simulink model "snb_bc"  (R2012b)
settings: Solver=FixedStepDiscrete  SolverMode=SingleTasking  StartTime=0.0  StopTime=10000  RelTol=1e-3
undefined symbols (not defined in the file): Down, pfb_coeff_gen_calc, Up
libraries: xbsIndex_r4 x19640, casper_library_misc x44, casper_library_delays x18, casper_library_communications x8, xps_library x3
(part 49 of 163)

== system snb_bc/mix_dec_fir/mixer/dds ==
  lo_const0 : Subsystem  AncestorBlock=casper_library_downconverter/lo_const  mask(lo_const){n_bits=10, phase=0}
      mask prompts: n_bits "Output Bitwidth"; phase "Phase (0 to 2*pi)"
      mask help:
      | Generates a complex constant associated with the
      | phase supplied as a parameter.
      mask init:
      | lo_const_init(gcb, ...
      |     'n_bits', n_bits, ...
      |     'phase', phase);
      mask Help: eval('xlWeb(''http://casper.berkeley.edu/wiki/Lo_const'')')
  lo_const1 : Subsystem  AncestorBlock=casper_library_downconverter/lo_const  mask(lo_const){n_bits=10, phase=1.5708}
      mask prompts: n_bits "Output Bitwidth"; phase "Phase (0 to 2*pi)"
      mask help:
      | Generates a complex constant associated with the
      | phase supplied as a parameter.
      mask init:
      | lo_const_init(gcb, ...
      |     'n_bits', n_bits, ...
      |     'phase', phase);
      mask Help: eval('xlWeb(''http://casper.berkeley.edu/wiki/Lo_const'')')
  lo_const2 : Subsystem  AncestorBlock=casper_library_downconverter/lo_const  mask(lo_const){n_bits=10, phase=3.1416}
      mask prompts: n_bits "Output Bitwidth"; phase "Phase (0 to 2*pi)"
      mask help:
      | Generates a complex constant associated with the
      | phase supplied as a parameter.
      mask init:
      | lo_const_init(gcb, ...
      |     'n_bits', n_bits, ...
      |     'phase', phase);
      mask Help: eval('xlWeb(''http://casper.berkeley.edu/wiki/Lo_const'')')
  lo_const3 : Subsystem  AncestorBlock=casper_library_downconverter/lo_const  mask(lo_const){n_bits=10, phase=4.7124}
      mask prompts: n_bits "Output Bitwidth"; phase "Phase (0 to 2*pi)"
      mask help:
      | Generates a complex constant associated with the
      | phase supplied as a parameter.
      mask init:
      | lo_const_init(gcb, ...
      |     'n_bits', n_bits, ...
      |     'phase', phase);
      mask Help: eval('xlWeb(''http://casper.berkeley.edu/wiki/Lo_const'')')
  lo_const4 : Subsystem  AncestorBlock=casper_library_downconverter/lo_const  mask(lo_const){n_bits=10, phase=6.2832}
      mask prompts: n_bits "Output Bitwidth"; phase "Phase (0 to 2*pi)"
      mask help:
      | Generates a complex constant associated with the
      | phase supplied as a parameter.
      mask init:
      | lo_const_init(gcb, ...
      |     'n_bits', n_bits, ...
      |     'phase', phase);
      mask Help: eval('xlWeb(''http://casper.berkeley.edu/wiki/Lo_const'')')
  lo_const5 : Subsystem  AncestorBlock=casper_library_downconverter/lo_const  mask(lo_const){n_bits=10, phase=7.854}
      mask prompts: n_bits "Output Bitwidth"; phase "Phase (0 to 2*pi)"
      mask help:
      | Generates a complex constant associated with the
      | phase supplied as a parameter.
      mask init:
      | lo_const_init(gcb, ...
      |     'n_bits', n_bits, ...
      |     'phase', phase);
      mask Help: eval('xlWeb(''http://casper.berkeley.edu/wiki/Lo_const'')')
  lo_const6 : Subsystem  AncestorBlock=casper_library_downconverter/lo_const  mask(lo_const){n_bits=10, phase=9.4248}
      mask prompts: n_bits "Output Bitwidth"; phase "Phase (0 to 2*pi)"
      mask help:
      | Generates a complex constant associated with the
      | phase supplied as a parameter.
      mask init:
      | lo_const_init(gcb, ...
      |     'n_bits', n_bits, ...
      |     'phase', phase);
      mask Help: eval('xlWeb(''http://casper.berkeley.edu/wiki/Lo_const'')')
  lo_const7 : Subsystem  AncestorBlock=casper_library_downconverter/lo_const  mask(lo_const){n_bits=10, phase=10.9956}
      mask prompts: n_bits "Output Bitwidth"; phase "Phase (0 to 2*pi)"
      mask help:
      | Generates a complex constant associated with the
      | phase supplied as a parameter.
      mask init:
      | lo_const_init(gcb, ...
      |     'n_bits', n_bits, ...
      |     'phase', phase);
      mask Help: eval('xlWeb(''http://casper.berkeley.edu/wiki/Lo_const'')')
  sin0 : Outport
  cos0 : Outport  Port=2
  sin1 : Outport  Port=3
  cos1 : Outport  Port=4
  sin2 : Outport  Port=5
  cos2 : Outport  Port=6
  sin3 : Outport  Port=7
  cos3 : Outport  Port=8
  sin4 : Outport  Port=9
  cos4 : Outport  Port=10
  sin5 : Outport  Port=11
  cos5 : Outport  Port=12
  sin6 : Outport  Port=13
  cos6 : Outport  Port=14
  sin7 : Outport  Port=15
  cos7 : Outport  Port=16
  wires:
  lo_const0/1(sin) -> sin0/1
  lo_const0/2(cos) -> cos0/1
  lo_const1/1(sin) -> sin1/1
  lo_const1/2(cos) -> cos1/1
  lo_const2/1(sin) -> sin2/1
  lo_const2/2(cos) -> cos2/1
  lo_const3/1(sin) -> sin3/1
  lo_const3/2(cos) -> cos3/1
  lo_const4/1(sin) -> sin4/1
  lo_const4/2(cos) -> cos4/1
  lo_const5/1(sin) -> sin5/1
  lo_const5/2(cos) -> cos5/1
  lo_const6/1(sin) -> sin6/1
  lo_const6/2(cos) -> cos6/1
  lo_const7/1(sin) -> sin7/1
  lo_const7/2(cos) -> cos7/1

== system snb_bc/mix_dec_fir/mixer/rcmult1 ==
  d : Inport
  sin : Inport  Port=2
  cos : Inport  Port=3
  Mult0 : xbsIndex_r4/Mult  precision=Full  arith_type="Signed  (2's comp)"  n_bits=8  bin_pt=2  quantization=Truncate  overflow=Wrap  en=off  latency=latency  dbl_ovrd=off  use_behavioral_HDL=off  opt=Speed  use_embedded=on  optimum_pipeline=off  pipeline=on  use_rpm=off  placement_style=Rectangular shape  block_type=mult
  Mult1 : xbsIndex_r4/Mult  precision=Full  arith_type="Signed  (2's comp)"  n_bits=8  bin_pt=2  quantization=Truncate  overflow=Wrap  en=off  latency=latency  dbl_ovrd=off  use_behavioral_HDL=off  opt=Speed  use_embedded=on  optimum_pipeline=off  pipeline=on  use_rpm=off  placement_style=Rectangular shape  block_type=mult
  real : Outport
  imag : Outport  Port=2
  wires:
  cos/1 -> Mult0/2
  sin/1 -> Mult1/2
  d/1 -> Mult1/1, Mult0/1
  Mult0/1 -> real/1
  Mult1/1 -> imag/1

== system snb_bc/mix_dec_fir/mixer/rcmult2 ==
  d : Inport
  sin : Inport  Port=2
  cos : Inport  Port=3
  Mult0 : xbsIndex_r4/Mult  precision=Full  arith_type="Signed  (2's comp)"  n_bits=8  bin_pt=2  quantization=Truncate  overflow=Wrap  en=off  latency=latency  dbl_ovrd=off  use_behavioral_HDL=off  opt=Speed  use_embedded=on  optimum_pipeline=off  pipeline=on  use_rpm=off  placement_style=Rectangular shape  block_type=mult
  Mult1 : xbsIndex_r4/Mult  precision=Full  arith_type="Signed  (2's comp)"  n_bits=8  bin_pt=2  quantization=Truncate  overflow=Wrap  en=off  latency=latency  dbl_ovrd=off  use_behavioral_HDL=off  opt=Speed  use_embedded=on  optimum_pipeline=off  pipeline=on  use_rpm=off  placement_style=Rectangular shape  block_type=mult
  real : Outport
  imag : Outport  Port=2
  wires:
  cos/1 -> Mult0/2
  sin/1 -> Mult1/2
  d/1 -> Mult1/1, Mult0/1
  Mult0/1 -> real/1
  Mult1/1 -> imag/1

== system snb_bc/mix_dec_fir/mixer/rcmult3 ==
  d : Inport
  sin : Inport  Port=2
  cos : Inport  Port=3
  Mult0 : xbsIndex_r4/Mult  precision=Full  arith_type="Signed  (2's comp)"  n_bits=8  bin_pt=2  quantization=Truncate  overflow=Wrap  en=off  latency=latency  dbl_ovrd=off  use_behavioral_HDL=off  opt=Speed  use_embedded=on  optimum_pipeline=off  pipeline=on  use_rpm=off  placement_style=Rectangular shape  block_type=mult
  Mult1 : xbsIndex_r4/Mult  precision=Full  arith_type="Signed  (2's comp)"  n_bits=8  bin_pt=2  quantization=Truncate  overflow=Wrap  en=off  latency=latency  dbl_ovrd=off  use_behavioral_HDL=off  opt=Speed  use_embedded=on  optimum_pipeline=off  pipeline=on  use_rpm=off  placement_style=Rectangular shape  block_type=mult
  real : Outport
  imag : Outport  Port=2
  wires:
  cos/1 -> Mult0/2
  sin/1 -> Mult1/2
  d/1 -> Mult1/1, Mult0/1
  Mult0/1 -> real/1
  Mult1/1 -> imag/1

== system snb_bc/mix_dec_fir/mixer/rcmult4 ==
  d : Inport
  sin : Inport  Port=2
  cos : Inport  Port=3
  Mult0 : xbsIndex_r4/Mult  precision=Full  arith_type="Signed  (2's comp)"  n_bits=8  bin_pt=2  quantization=Truncate  overflow=Wrap  en=off  latency=latency  dbl_ovrd=off  use_behavioral_HDL=off  opt=Speed  use_embedded=on  optimum_pipeline=off  pipeline=on  use_rpm=off  placement_style=Rectangular shape  block_type=mult
  Mult1 : xbsIndex_r4/Mult  precision=Full  arith_type="Signed  (2's comp)"  n_bits=8  bin_pt=2  quantization=Truncate  overflow=Wrap  en=off  latency=latency  dbl_ovrd=off  use_behavioral_HDL=off  opt=Speed  use_embedded=on  optimum_pipeline=off  pipeline=on  use_rpm=off  placement_style=Rectangular shape  block_type=mult
  real : Outport
  imag : Outport  Port=2
  wires:
  cos/1 -> Mult0/2
  sin/1 -> Mult1/2
  d/1 -> Mult1/1, Mult0/1
  Mult0/1 -> real/1
  Mult1/1 -> imag/1

== system snb_bc/mix_dec_fir/mixer/rcmult5 ==
  d : Inport
  sin : Inport  Port=2
  cos : Inport  Port=3
  Mult0 : xbsIndex_r4/Mult  precision=Full  arith_type="Signed  (2's comp)"  n_bits=8  bin_pt=2  quantization=Truncate  overflow=Wrap  en=off  latency=latency  dbl_ovrd=off  use_behavioral_HDL=off  opt=Speed  use_embedded=on  optimum_pipeline=off  pipeline=on  use_rpm=off  placement_style=Rectangular shape  block_type=mult
  Mult1 : xbsIndex_r4/Mult  precision=Full  arith_type="Signed  (2's comp)"  n_bits=8  bin_pt=2  quantization=Truncate  overflow=Wrap  en=off  latency=latency  dbl_ovrd=off  use_behavioral_HDL=off  opt=Speed  use_embedded=on  optimum_pipeline=off  pipeline=on  use_rpm=off  placement_style=Rectangular shape  block_type=mult
  real : Outport
  imag : Outport  Port=2
  wires:
  cos/1 -> Mult0/2
  sin/1 -> Mult1/2
  d/1 -> Mult1/1, Mult0/1
  Mult0/1 -> real/1
  Mult1/1 -> imag/1

== system snb_bc/mix_dec_fir/mixer/rcmult6 ==
  d : Inport
  sin : Inport  Port=2
  cos : Inport  Port=3
  Mult0 : xbsIndex_r4/Mult  precision=Full  arith_type="Signed  (2's comp)"  n_bits=8  bin_pt=2  quantization=Truncate  overflow=Wrap  en=off  latency=latency  dbl_ovrd=off  use_behavioral_HDL=off  opt=Speed  use_embedded=on  optimum_pipeline=off  pipeline=on  use_rpm=off  placement_style=Rectangular shape  block_type=mult
  Mult1 : xbsIndex_r4/Mult  precision=Full  arith_type="Signed  (2's comp)"  n_bits=8  bin_pt=2  quantization=Truncate  overflow=Wrap  en=off  latency=latency  dbl_ovrd=off  use_behavioral_HDL=off  opt=Speed  use_embedded=on  optimum_pipeline=off  pipeline=on  use_rpm=off  placement_style=Rectangular shape  block_type=mult
  real : Outport
  imag : Outport  Port=2
  wires:
  cos/1 -> Mult0/2
  sin/1 -> Mult1/2
  d/1 -> Mult1/1, Mult0/1
  Mult0/1 -> real/1
  Mult1/1 -> imag/1

== system snb_bc/mix_dec_fir/mixer/rcmult7 ==
  d : Inport
  sin : Inport  Port=2
  cos : Inport  Port=3
  Mult0 : xbsIndex_r4/Mult  precision=Full  arith_type="Signed  (2's comp)"  n_bits=8  bin_pt=2  quantization=Truncate  overflow=Wrap  en=off  latency=latency  dbl_ovrd=off  use_behavioral_HDL=off  opt=Speed  use_embedded=on  optimum_pipeline=off  pipeline=on  use_rpm=off  placement_style=Rectangular shape  block_type=mult
  Mult1 : xbsIndex_r4/Mult  precision=Full  arith_type="Signed  (2's comp)"  n_bits=8  bin_pt=2  quantization=Truncate  overflow=Wrap  en=off  latency=latency  dbl_ovrd=off  use_behavioral_HDL=off  opt=Speed  use_embedded=on  optimum_pipeline=off  pipeline=on  use_rpm=off  placement_style=Rectangular shape  block_type=mult
  real : Outport
  imag : Outport  Port=2
  wires:
  cos/1 -> Mult0/2
  sin/1 -> Mult1/2
  d/1 -> Mult1/1, Mult0/1
  Mult0/1 -> real/1
  Mult1/1 -> imag/1

== system snb_bc/mix_dec_fir/mixer/rcmult8 ==
  d : Inport
  sin : Inport  Port=2
  cos : Inport  Port=3
  Mult0 : xbsIndex_r4/Mult  precision=Full  arith_type="Signed  (2's comp)"  n_bits=8  bin_pt=2  quantization=Truncate  overflow=Wrap  en=off  latency=latency  dbl_ovrd=off  use_behavioral_HDL=off  opt=Speed  use_embedded=on  optimum_pipeline=off  pipeline=on  use_rpm=off  placement_style=Rectangular shape  block_type=mult
  Mult1 : xbsIndex_r4/Mult  precision=Full  arith_type="Signed  (2's comp)"  n_bits=8  bin_pt=2  quantization=Truncate  overflow=Wrap  en=off  latency=latency  dbl_ovrd=off  use_behavioral_HDL=off  opt=Speed  use_embedded=on  optimum_pipeline=off  pipeline=on  use_rpm=off  placement_style=Rectangular shape  block_type=mult
  real : Outport
  imag : Outport  Port=2
  wires:
  cos/1 -> Mult0/2
  sin/1 -> Mult1/2
  d/1 -> Mult1/1, Mult0/1
  Mult0/1 -> real/1
  Mult1/1 -> imag/1

== system snb_bc/mix_dec_fir/mixer1/dds ==
  lo_const0 : Subsystem  AncestorBlock=casper_library_downconverter/lo_const  mask(lo_const){n_bits=10, phase=0}
      mask prompts: n_bits "Output Bitwidth"; phase "Phase (0 to 2*pi)"
      mask help:
      | Generates a complex constant associated with the
      | phase supplied as a parameter.
      mask init:
      | lo_const_init(gcb, ...
      |     'n_bits', n_bits, ...
      |     'phase', phase);
      mask Help: eval('xlWeb(''http://casper.berkeley.edu/wiki/Lo_const'')')
  lo_const1 : Subsystem  AncestorBlock=casper_library_downconverter/lo_const  mask(lo_const){n_bits=10, phase=1.5708}
      mask prompts: n_bits "Output Bitwidth"; phase "Phase (0 to 2*pi)"
      mask help:
      | Generates a complex constant associated with the
      | phase supplied as a parameter.
      mask init:
      | lo_const_init(gcb, ...
      |     'n_bits', n_bits, ...
      |     'phase', phase);
      mask Help: eval('xlWeb(''http://casper.berkeley.edu/wiki/Lo_const'')')
  lo_const2 : Subsystem  AncestorBlock=casper_library_downconverter/lo_const  mask(lo_const){n_bits=10, phase=3.1416}
      mask prompts: n_bits "Output Bitwidth"; phase "Phase (0 to 2*pi)"
      mask help:
      | Generates a complex constant associated with the
      | phase supplied as a parameter.
      mask init:
      | lo_const_init(gcb, ...
      |     'n_bits', n_bits, ...
      |     'phase', phase);
      mask Help: eval('xlWeb(''http://casper.berkeley.edu/wiki/Lo_const'')')
  lo_const3 : Subsystem  AncestorBlock=casper_library_downconverter/lo_const  mask(lo_const){n_bits=10, phase=4.7124}
      mask prompts: n_bits "Output Bitwidth"; phase "Phase (0 to 2*pi)"
      mask help:
      | Generates a complex constant associated with the
      | phase supplied as a parameter.
      mask init:
      | lo_const_init(gcb, ...
      |     'n_bits', n_bits, ...
      |     'phase', phase);
      mask Help: eval('xlWeb(''http://casper.berkeley.edu/wiki/Lo_const'')')
  lo_const4 : Subsystem  AncestorBlock=casper_library_downconverter/lo_const  mask(lo_const){n_bits=10, phase=6.2832}
      mask prompts: n_bits "Output Bitwidth"; phase "Phase (0 to 2*pi)"
      mask help:
      | Generates a complex constant associated with the
      | phase supplied as a parameter.
      mask init:
      | lo_const_init(gcb, ...
      |     'n_bits', n_bits, ...
      |     'phase', phase);
      mask Help: eval('xlWeb(''http://casper.berkeley.edu/wiki/Lo_const'')')
  lo_const5 : Subsystem  AncestorBlock=casper_library_downconverter/lo_const  mask(lo_const){n_bits=10, phase=7.854}
      mask prompts: n_bits "Output Bitwidth"; phase "Phase (0 to 2*pi)"
      mask help:
      | Generates a complex constant associated with the
      | phase supplied as a parameter.
      mask init:
      | lo_const_init(gcb, ...
      |     'n_bits', n_bits, ...
      |     'phase', phase);
      mask Help: eval('xlWeb(''http://casper.berkeley.edu/wiki/Lo_const'')')
  lo_const6 : Subsystem  AncestorBlock=casper_library_downconverter/lo_const  mask(lo_const){n_bits=10, phase=9.4248}
      mask prompts: n_bits "Output Bitwidth"; phase "Phase (0 to 2*pi)"
      mask help:
      | Generates a complex constant associated with the
      | phase supplied as a parameter.
      mask init:
      | lo_const_init(gcb, ...
      |     'n_bits', n_bits, ...
      |     'phase', phase);
      mask Help: eval('xlWeb(''http://casper.berkeley.edu/wiki/Lo_const'')')
  lo_const7 : Subsystem  AncestorBlock=casper_library_downconverter/lo_const  mask(lo_const){n_bits=10, phase=10.9956}
      mask prompts: n_bits "Output Bitwidth"; phase "Phase (0 to 2*pi)"
      mask help:
      | Generates a complex constant associated with the
      | phase supplied as a parameter.
      mask init:
      | lo_const_init(gcb, ...
      |     'n_bits', n_bits, ...
      |     'phase', phase);
      mask Help: eval('xlWeb(''http://casper.berkeley.edu/wiki/Lo_const'')')
  sin0 : Outport
  cos0 : Outport  Port=2
  sin1 : Outport  Port=3
  cos1 : Outport  Port=4
  sin2 : Outport  Port=5
  cos2 : Outport  Port=6
  sin3 : Outport  Port=7
  cos3 : Outport  Port=8
  sin4 : Outport  Port=9
  cos4 : Outport  Port=10
  sin5 : Outport  Port=11
  cos5 : Outport  Port=12
  sin6 : Outport  Port=13
  cos6 : Outport  Port=14
  sin7 : Outport  Port=15
  cos7 : Outport  Port=16
  wires:
  lo_const7/2(cos) -> cos7/1
  lo_const7/1(sin) -> sin7/1
  lo_const6/2(cos) -> cos6/1
  lo_const6/1(sin) -> sin6/1
  lo_const5/2(cos) -> cos5/1
  lo_const5/1(sin) -> sin5/1
  lo_const4/2(cos) -> cos4/1
  lo_const4/1(sin) -> sin4/1
  lo_const3/2(cos) -> cos3/1
  lo_const3/1(sin) -> sin3/1
  lo_const2/2(cos) -> cos2/1
  lo_const2/1(sin) -> sin2/1
  lo_const1/2(cos) -> cos1/1
  lo_const1/1(sin) -> sin1/1
  lo_const0/2(cos) -> cos0/1
  lo_const0/1(sin) -> sin0/1

== system snb_bc/mix_dec_fir/mixer1/rcmult1 ==
  d : Inport
  sin : Inport  Port=2
  cos : Inport  Port=3
  Mult0 : xbsIndex_r4/Mult  precision=Full  arith_type="Signed  (2's comp)"  n_bits=8  bin_pt=2  quantization=Truncate  overflow=Wrap  en=off  latency=latency  dbl_ovrd=off  use_behavioral_HDL=off  opt=Speed  use_embedded=on  optimum_pipeline=off  pipeline=on  use_rpm=off  placement_style=Rectangular shape  block_type=mult
  Mult1 : xbsIndex_r4/Mult  precision=Full  arith_type="Signed  (2's comp)"  n_bits=8  bin_pt=2  quantization=Truncate  overflow=Wrap  en=off  latency=latency  dbl_ovrd=off  use_behavioral_HDL=off  opt=Speed  use_embedded=on  optimum_pipeline=off  pipeline=on  use_rpm=off  placement_style=Rectangular shape  block_type=mult
  real : Outport
  imag : Outport  Port=2
  wires:
  Mult1/1 -> imag/1
  Mult0/1 -> real/1
  d/1 -> Mult0/1, Mult1/1
  sin/1 -> Mult1/2
  cos/1 -> Mult0/2

== system snb_bc/mix_dec_fir/mixer1/rcmult2 ==
  d : Inport
  sin : Inport  Port=2
  cos : Inport  Port=3
  Mult0 : xbsIndex_r4/Mult  precision=Full  arith_type="Signed  (2's comp)"  n_bits=8  bin_pt=2  quantization=Truncate  overflow=Wrap  en=off  latency=latency  dbl_ovrd=off  use_behavioral_HDL=off  opt=Speed  use_embedded=on  optimum_pipeline=off  pipeline=on  use_rpm=off  placement_style=Rectangular shape  block_type=mult
  Mult1 : xbsIndex_r4/Mult  precision=Full  arith_type="Signed  (2's comp)"  n_bits=8  bin_pt=2  quantization=Truncate  overflow=Wrap  en=off  latency=latency  dbl_ovrd=off  use_behavioral_HDL=off  opt=Speed  use_embedded=on  optimum_pipeline=off  pipeline=on  use_rpm=off  placement_style=Rectangular shape  block_type=mult
  real : Outport
  imag : Outport  Port=2
  wires:
  Mult1/1 -> imag/1
  Mult0/1 -> real/1
  d/1 -> Mult0/1, Mult1/1
  sin/1 -> Mult1/2
  cos/1 -> Mult0/2

== system snb_bc/mix_dec_fir/mixer1/rcmult3 ==
  d : Inport
  sin : Inport  Port=2
  cos : Inport  Port=3
  Mult0 : xbsIndex_r4/Mult  precision=Full  arith_type="Signed  (2's comp)"  n_bits=8  bin_pt=2  quantization=Truncate  overflow=Wrap  en=off  latency=latency  dbl_ovrd=off  use_behavioral_HDL=off  opt=Speed  use_embedded=on  optimum_pipeline=off  pipeline=on  use_rpm=off  placement_style=Rectangular shape  block_type=mult
  Mult1 : xbsIndex_r4/Mult  precision=Full  arith_type="Signed  (2's comp)"  n_bits=8  bin_pt=2  quantization=Truncate  overflow=Wrap  en=off  latency=latency  dbl_ovrd=off  use_behavioral_HDL=off  opt=Speed  use_embedded=on  optimum_pipeline=off  pipeline=on  use_rpm=off  placement_style=Rectangular shape  block_type=mult
  real : Outport
  imag : Outport  Port=2
  wires:
  Mult1/1 -> imag/1
  Mult0/1 -> real/1
  d/1 -> Mult0/1, Mult1/1
  sin/1 -> Mult1/2
  cos/1 -> Mult0/2

== system snb_bc/mix_dec_fir/mixer1/rcmult4 ==
  d : Inport
  sin : Inport  Port=2
  cos : Inport  Port=3
  Mult0 : xbsIndex_r4/Mult  precision=Full  arith_type="Signed  (2's comp)"  n_bits=8  bin_pt=2  quantization=Truncate  overflow=Wrap  en=off  latency=latency  dbl_ovrd=off  use_behavioral_HDL=off  opt=Speed  use_embedded=on  optimum_pipeline=off  pipeline=on  use_rpm=off  placement_style=Rectangular shape  block_type=mult
  Mult1 : xbsIndex_r4/Mult  precision=Full  arith_type="Signed  (2's comp)"  n_bits=8  bin_pt=2  quantization=Truncate  overflow=Wrap  en=off  latency=latency  dbl_ovrd=off  use_behavioral_HDL=off  opt=Speed  use_embedded=on  optimum_pipeline=off  pipeline=on  use_rpm=off  placement_style=Rectangular shape  block_type=mult
  real : Outport
  imag : Outport  Port=2
  wires:
  Mult1/1 -> imag/1
  Mult0/1 -> real/1
  d/1 -> Mult0/1, Mult1/1
  sin/1 -> Mult1/2
  cos/1 -> Mult0/2

== system snb_bc/mix_dec_fir/mixer1/rcmult5 ==
  d : Inport
  sin : Inport  Port=2
  cos : Inport  Port=3
  Mult0 : xbsIndex_r4/Mult  precision=Full  arith_type="Signed  (2's comp)"  n_bits=8  bin_pt=2  quantization=Truncate  overflow=Wrap  en=off  latency=latency  dbl_ovrd=off  use_behavioral_HDL=off  opt=Speed  use_embedded=on  optimum_pipeline=off  pipeline=on  use_rpm=off  placement_style=Rectangular shape  block_type=mult
  Mult1 : xbsIndex_r4/Mult  precision=Full  arith_type="Signed  (2's comp)"  n_bits=8  bin_pt=2  quantization=Truncate  overflow=Wrap  en=off  latency=latency  dbl_ovrd=off  use_behavioral_HDL=off  opt=Speed  use_embedded=on  optimum_pipeline=off  pipeline=on  use_rpm=off  placement_style=Rectangular shape  block_type=mult
  real : Outport
  imag : Outport  Port=2
  wires:
  Mult1/1 -> imag/1
  Mult0/1 -> real/1
  d/1 -> Mult0/1, Mult1/1
  sin/1 -> Mult1/2
  cos/1 -> Mult0/2

== system snb_bc/mix_dec_fir/mixer1/rcmult6 ==
  d : Inport
  sin : Inport  Port=2
  cos : Inport  Port=3
  Mult0 : xbsIndex_r4/Mult  precision=Full  arith_type="Signed  (2's comp)"  n_bits=8  bin_pt=2  quantization=Truncate  overflow=Wrap  en=off  latency=latency  dbl_ovrd=off  use_behavioral_HDL=off  opt=Speed  use_embedded=on  optimum_pipeline=off  pipeline=on  use_rpm=off  placement_style=Rectangular shape  block_type=mult
  Mult1 : xbsIndex_r4/Mult  precision=Full  arith_type="Signed  (2's comp)"  n_bits=8  bin_pt=2  quantization=Truncate  overflow=Wrap  en=off  latency=latency  dbl_ovrd=off  use_behavioral_HDL=off  opt=Speed  use_embedded=on  optimum_pipeline=off  pipeline=on  use_rpm=off  placement_style=Rectangular shape  block_type=mult
  real : Outport
  imag : Outport  Port=2
  wires:
  Mult1/1 -> imag/1
  Mult0/1 -> real/1
  d/1 -> Mult0/1, Mult1/1
  sin/1 -> Mult1/2
  cos/1 -> Mult0/2

== system snb_bc/mix_dec_fir/mixer1/rcmult7 ==
  d : Inport
  sin : Inport  Port=2
  cos : Inport  Port=3
  Mult0 : xbsIndex_r4/Mult  precision=Full  arith_type="Signed  (2's comp)"  n_bits=8  bin_pt=2  quantization=Truncate  overflow=Wrap  en=off  latency=latency  dbl_ovrd=off  use_behavioral_HDL=off  opt=Speed  use_embedded=on  optimum_pipeline=off  pipeline=on  use_rpm=off  placement_style=Rectangular shape  block_type=mult
  Mult1 : xbsIndex_r4/Mult  precision=Full  arith_type="Signed  (2's comp)"  n_bits=8  bin_pt=2  quantization=Truncate  overflow=Wrap  en=off  latency=latency  dbl_ovrd=off  use_behavioral_HDL=off  opt=Speed  use_embedded=on  optimum_pipeline=off  pipeline=on  use_rpm=off  placement_style=Rectangular shape  block_type=mult
  real : Outport
  imag : Outport  Port=2
  wires:
  Mult1/1 -> imag/1
  Mult0/1 -> real/1
  d/1 -> Mult0/1, Mult1/1
  sin/1 -> Mult1/2
  cos/1 -> Mult0/2

== system snb_bc/mix_dec_fir/mixer1/rcmult8 ==
  d : Inport
  sin : Inport  Port=2
  cos : Inport  Port=3
  Mult0 : xbsIndex_r4/Mult  precision=Full  arith_type="Signed  (2's comp)"  n_bits=8  bin_pt=2  quantization=Truncate  overflow=Wrap  en=off  latency=latency  dbl_ovrd=off  use_behavioral_HDL=off  opt=Speed  use_embedded=on  optimum_pipeline=off  pipeline=on  use_rpm=off  placement_style=Rectangular shape  block_type=mult
  Mult1 : xbsIndex_r4/Mult  precision=Full  arith_type="Signed  (2's comp)"  n_bits=8  bin_pt=2  quantization=Truncate  overflow=Wrap  en=off  latency=latency  dbl_ovrd=off  use_behavioral_HDL=off  opt=Speed  use_embedded=on  optimum_pipeline=off  pipeline=on  use_rpm=off  placement_style=Rectangular shape  block_type=mult
  real : Outport
  imag : Outport  Port=2
  wires:
  Mult1/1 -> imag/1
  Mult0/1 -> real/1
  d/1 -> Mult0/1, Mult1/1
  sin/1 -> Mult1/2
  cos/1 -> Mult0/2

== system snb_bc/pack/spead_pack/edge_detect1 ==
  in : Inport
  Delay : xbsIndex_r4/Delay  rst=off  infoeditControl=Selection of Reset will increase slice count due to use of real FFs and instead of SRLs  en=off  latency=1  dbl_ovrd=off  reg_retiming=off  block_type=delay
      settings: xl_area=[0, 0, 0, 0, 0, 0, 0]
  Inverter : xbsIndex_r4/Inverter  en=off  latency=0  dbl_ovrd=off  block_type=inv
      settings: xl_area=[0, 0, 0, 0, 0, 0, 0]
  edge_op : xbsIndex_r4/Logical  logical_function=NOR  inputs=2  en=off  latency=0  precision=Full  arith_type=Unsigned  n_bits=8  bin_pt=2  align_bp=on  dbl_ovrd=off  block_type=logical
      settings: xl_area=[0, 0, 0, 0, 0, 0, 0]
  out : Outport
  wires:
  Delay/1 -> edge_op/2
  in/1 -> Delay/1, Inverter/1
  edge_op/1 -> out/1
  Inverter/1 -> edge_op/1

== system snb_bc/pack/spead_pack/edge_detect2 ==
  in : Inport
  Delay : xbsIndex_r4/Delay  rst=off  infoeditControl=Selection of Reset will increase slice count due to use of real FFs and instead of SRLs  en=off  latency=1  dbl_ovrd=off  reg_retiming=off  block_type=delay
      settings: xl_area=[0, 0, 0, 0, 0, 0, 0]
  Inverter : xbsIndex_r4/Inverter  en=off  latency=0  dbl_ovrd=off  block_type=inv
      settings: xl_area=[0, 0, 0, 0, 0, 0, 0]
  edge_op : xbsIndex_r4/Logical  logical_function=NOR  inputs=2  en=off  latency=0  precision=Full  arith_type=Unsigned  n_bits=8  bin_pt=2  align_bp=on  dbl_ovrd=off  block_type=logical
      settings: xl_area=[0, 0, 0, 0, 0, 0, 0]
  out : Outport
  wires:
  Inverter/1 -> edge_op/1
  edge_op/1 -> out/1
  in/1 -> Inverter/1, Delay/1
  Delay/1 -> edge_op/2

== system snb_bc/pack/spead_pack1/edge_detect1 ==
  in : Inport
  Delay : xbsIndex_r4/Delay  rst=off  infoeditControl=Selection of Reset will increase slice count due to use of real FFs and instead of SRLs  en=off  latency=1  dbl_ovrd=off  reg_retiming=off  block_type=delay
      settings: xl_area=[0, 0, 0, 0, 0, 0, 0]
  Inverter : xbsIndex_r4/Inverter  en=off  latency=0  dbl_ovrd=off  block_type=inv
      settings: xl_area=[0, 0, 0, 0, 0, 0, 0]
  edge_op : xbsIndex_r4/Logical  logical_function=NOR  inputs=2  en=off  latency=0  precision=Full  arith_type=Unsigned  n_bits=8  bin_pt=2  align_bp=on  dbl_ovrd=off  block_type=logical
      settings: xl_area=[0, 0, 0, 0, 0, 0, 0]
  out : Outport
  wires:
  Inverter/1 -> edge_op/1
  edge_op/1 -> out/1
  in/1 -> Inverter/1, Delay/1
  Delay/1 -> edge_op/2

== system snb_bc/pack/spead_pack1/edge_detect2 ==
  in : Inport
  Delay : xbsIndex_r4/Delay  rst=off  infoeditControl=Selection of Reset will increase slice count due to use of real FFs and instead of SRLs  en=off  latency=1  dbl_ovrd=off  reg_retiming=off  block_type=delay
      settings: xl_area=[0, 0, 0, 0, 0, 0, 0]
  Inverter : xbsIndex_r4/Inverter  en=off  latency=0  dbl_ovrd=off  block_type=inv
      settings: xl_area=[0, 0, 0, 0, 0, 0, 0]
  edge_op : xbsIndex_r4/Logical  logical_function=NOR  inputs=2  en=off  latency=0  precision=Full  arith_type=Unsigned  n_bits=8  bin_pt=2  align_bp=on  dbl_ovrd=off  block_type=logical
      settings: xl_area=[0, 0, 0, 0, 0, 0, 0]
  out : Outport
  wires:
  Delay/1 -> edge_op/2
  in/1 -> Delay/1, Inverter/1
  edge_op/1 -> out/1
  Inverter/1 -> edge_op/1

== system snb_bc/pack/spead_pack2/edge_detect1 ==
  in : Inport
  Delay : xbsIndex_r4/Delay  rst=off  infoeditControl=Selection of Reset will increase slice count due to use of real FFs and instead of SRLs  en=off  latency=1  dbl_ovrd=off  reg_retiming=off  block_type=delay
      settings: xl_area=[0, 0, 0, 0, 0, 0, 0]
  Inverter : xbsIndex_r4/Inverter  en=off  latency=0  dbl_ovrd=off  block_type=inv
      settings: xl_area=[0, 0, 0, 0, 0, 0, 0]
  edge_op : xbsIndex_r4/Logical  logical_function=NOR  inputs=2  en=off  latency=0  precision=Full  arith_type=Unsigned  n_bits=8  bin_pt=2  align_bp=on  dbl_ovrd=off  block_type=logical
      settings: xl_area=[0, 0, 0, 0, 0, 0, 0]
  out : Outport
  wires:
  Delay/1 -> edge_op/2
  in/1 -> Delay/1, Inverter/1
  edge_op/1 -> out/1
  Inverter/1 -> edge_op/1

== system snb_bc/pack/spead_pack2/edge_detect2 ==
  in : Inport
  Delay : xbsIndex_r4/Delay  rst=off  infoeditControl=Selection of Reset will increase slice count due to use of real FFs and instead of SRLs  en=off  latency=1  dbl_ovrd=off  reg_retiming=off  block_type=delay
      settings: xl_area=[0, 0, 0, 0, 0, 0, 0]
  Inverter : xbsIndex_r4/Inverter  en=off  latency=0  dbl_ovrd=off  block_type=inv
      settings: xl_area=[0, 0, 0, 0, 0, 0, 0]
  edge_op : xbsIndex_r4/Logical  logical_function=NOR  inputs=2  en=off  latency=0  precision=Full  arith_type=Unsigned  n_bits=8  bin_pt=2  align_bp=on  dbl_ovrd=off  block_type=logical
      settings: xl_area=[0, 0, 0, 0, 0, 0, 0]
  out : Outport
  wires:
  Inverter/1 -> edge_op/1
  edge_op/1 -> out/1
  in/1 -> Inverter/1, Delay/1
  Delay/1 -> edge_op/2

== system snb_bc/pack/spead_pack3/edge_detect1 ==
  in : Inport
  Delay : xbsIndex_r4/Delay  rst=off  infoeditControl=Selection of Reset will increase slice count due to use of real FFs and instead of SRLs  en=off  latency=1  dbl_ovrd=off  reg_retiming=off  block_type=delay
      settings: xl_area=[0, 0, 0, 0, 0, 0, 0]
  Inverter : xbsIndex_r4/Inverter  en=off  latency=0  dbl_ovrd=off  block_type=inv
      settings: xl_area=[0, 0, 0, 0, 0, 0, 0]
  edge_op : xbsIndex_r4/Logical  logical_function=NOR  inputs=2  en=off  latency=0  precision=Full  arith_type=Unsigned  n_bits=8  bin_pt=2  align_bp=on  dbl_ovrd=off  block_type=logical
      settings: xl_area=[0, 0, 0, 0, 0, 0, 0]
  out : Outport
  wires:
  Inverter/1 -> edge_op/1
  edge_op/1 -> out/1
  in/1 -> Inverter/1, Delay/1
  Delay/1 -> edge_op/2

== system snb_bc/pack/spead_pack3/edge_detect2 ==
  in : Inport
  Delay : xbsIndex_r4/Delay  rst=off  infoeditControl=Selection of Reset will increase slice count due to use of real FFs and instead of SRLs  en=off  latency=1  dbl_ovrd=off  reg_retiming=off  block_type=delay
      settings: xl_area=[0, 0, 0, 0, 0, 0, 0]
  Inverter : xbsIndex_r4/Inverter  en=off  latency=0  dbl_ovrd=off  block_type=inv
      settings: xl_area=[0, 0, 0, 0, 0, 0, 0]
  edge_op : xbsIndex_r4/Logical  logical_function=NOR  inputs=2  en=off  latency=0  precision=Full  arith_type=Unsigned  n_bits=8  bin_pt=2  align_bp=on  dbl_ovrd=off  block_type=logical
      settings: xl_area=[0, 0, 0, 0, 0, 0, 0]
  out : Outport
  wires:
  Delay/1 -> edge_op/2
  in/1 -> Delay/1, Inverter/1
  edge_op/1 -> out/1
  Inverter/1 -> edge_op/1
